simulink model "cochons_optim"  (R2013b)
settings: Solver=ode45  StartTime=0  StopTime=12000  RelTol=1e-3
libraries: simulink x3
settings Model: TunableVars=p  TunableVarsStorageClass=Auto  Creator=ltraonou  LastModifiedBy=ltraonou
settings SolverCC: ShapePreserveControl=EnableAll
settings DataIOCC: FinalStateName=last_state  InitialState=last_state  LimitDataPoints=off  SaveFormat=StructureWithTime  SaveOutput=off  SaveTime=off
settings OptimizationCC: InlineParams=on
settings DebuggingCC: MultiTaskDSMMsg=warning  MultiTaskCondExecSysMsg=none
settings RTWCC: IncludeERTFirstTime=on

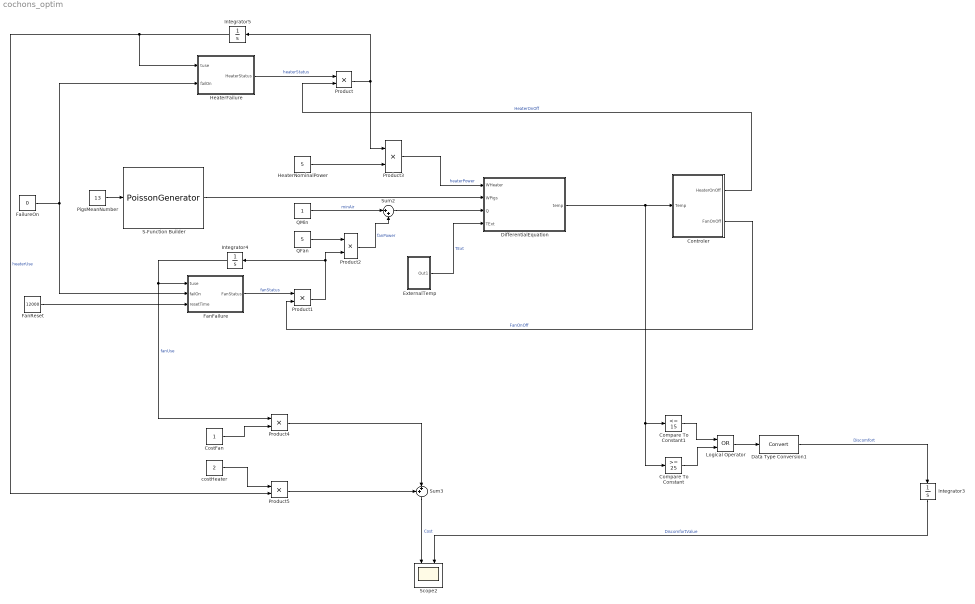
== system cochons_optim ==
  Compare To Constant : simulink/Logic and Bit Operations/Compare To Constant  relop=>=  const=25  OutDataTypeStr=boolean
  Compare To Constant1 : simulink/Logic and Bit Operations/Compare To Constant  relop=<=  const=15  OutDataTypeStr=boolean
  Controler : Subsystem
  CostFan : Constant
  Data Type Conversion1 : DataTypeConversion
  DifferentialEquation : Subsystem
  ExternalTemp : Subsystem
  FailureOn : Constant  Value=0
  FanFailure : Subsystem
  FanReset : Constant  Value=12000
  HeaterFailure : Subsystem
  HeaterNominalPower : Constant  Value=5
  Integrator3 : Integrator  InitialCondition=0.0001
  Integrator4 : Integrator
  Integrator5 : Integrator
  Logical Operator : Logic  Operator=OR  AllPortsSameDT=off  OutDataTypeStr=boolean
  PigsMeanNumber : Constant  Value=13
  Product{,1..5} (6 alike) : Product
  QFan : Constant  Value=5
  QMin : Constant
  S-Function Builder : S-Function  InitFcn=try, set_param(gcb,'FunctionName','PoissonGenerator'), end  FunctionName=PoissonGenerator  SFunctionModules=PoissonGenerator_wrapper  EnableBusSupport=off  mask(S-Function Builder){}
      mask help: Simulink:masks:SFunctionBuilder_MD
      mask init:
      | val = [[.9  0.75 0.75 1 1 .9 .9 1]',[1 1 0.75 0.75 .9 .9 1 .9]'];try , sys = get_param(gcb,'SfunBuilderFcnName');if isempty(sys), sys = get_param(gcb,'FunctionName'); end,catch, sys = get_param(gcb,'FunctionName'); end
      settings: CopyFcn=set_param(gcbh,'LinkStatus','none')  PreSaveFcn=try, set_param(gcb,'FunctionName','PoissonGenerator'), end  OpenFcn=sfunctionwizard(gcbh)
      mask Display: plot(val(:,1),val(:,2)),disp(sys), port_label('input',1,'lambda'), port_label('output',1,'y')
  Scope2 : Scope  NumInputPorts=2
      settings: YMin=0~0  YMax=7500~325
  Sum2 : Sum  Inputs=|++
  Sum3 : Sum  Inputs=++|
  costHeater : Constant  Value=2
  wires:
  QFan/1 -> Product2/1
  QMin/1 -> Sum2/1  "minAir"
  Product2/1 -> Sum2/2  "fanPower"
  Product3/1 -> DifferentialEquation/1(WHeater)  "heaterPower"
  HeaterNominalPower/1 -> Product3/2
  FanFailure/1(FanStatus) -> Product1/1  "fanStatus"
  HeaterFailure/1(HeaterStatus) -> Product/1  "heaterStatus"
  Controler/2(FanOnOff) -> Product1/2  "FanOnOff"
  Controler/1(HeaterOnOff) -> Product/2  "HeaterOnOff"
  Data Type Conversion1/1 -> Integrator3/1  "Discomfort"
  DifferentialEquation/1(temp) -> Controler/1(Temp), Compare To Constant/1, Compare To Constant1/1
  S-Function Builder/1 -> DifferentialEquation/2(WPigs)
  Sum2/1 -> DifferentialEquation/3(Q)
  PigsMeanNumber/1 -> S-Function Builder/1
  ExternalTemp/1(Out1) -> DifferentialEquation/4(TExt)  "TExt"
  Compare To Constant1/1 -> Logical Operator/1
  Compare To Constant/1 -> Logical Operator/2
  Logical Operator/1 -> Data Type Conversion1/1
  Product/1 -> Integrator5/1, Product3/1
  Product1/1 -> Product2/2, Integrator4/1
  FailureOn/1 -> HeaterFailure/2(failOn), FanFailure/2(failOn)
  FanReset/1 -> FanFailure/3(resetTime)
  Integrator3/1 -> Scope2/2  "DiscomfortValue"
  CostFan/1 -> Product4/2
  Product4/1 -> Sum3/2
  Sum3/1 -> Scope2/1  "Cost"
  Integrator4/1 -> Product4/1, FanFailure/1(tuse)  "fanUse"
  Integrator5/1 -> HeaterFailure/1(tuse), Product5/2  "heaterUse"
  costHeater/1 -> Product5/1
  Product5/1 -> Sum3/1

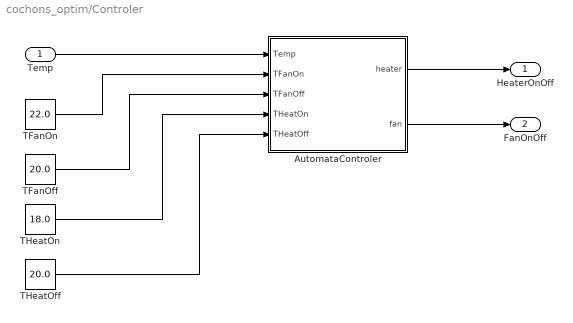
== system cochons_optim/Controler ==
  Temp : Inport
  AutomataControler : Stateflow chart  TreatAsAtomicUnit=on
  TFanOff : Constant  Value=20.0
  TFanOn : Constant  Value=22.0
  THeatOff : Constant  Value=20.0
  THeatOn : Constant  Value=18.0
  HeaterOnOff : Outport
  FanOnOff : Outport  Port=2
  wires:
  Temp/1 -> AutomataControler/1(Temp)
  TFanOn/1 -> AutomataControler/2(TFanOn)
  THeatOn/1 -> AutomataControler/4(THeatOn)
  THeatOff/1 -> AutomataControler/5(THeatOff)
  TFanOff/1 -> AutomataControler/3(TFanOff)
  AutomataControler/2(fan) -> FanOnOff/1
  AutomataControler/1(heater) -> HeaterOnOff/1

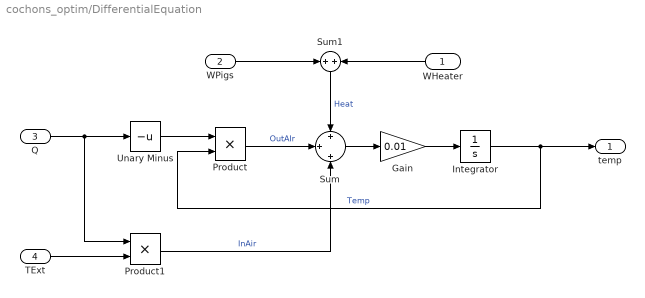
== system cochons_optim/DifferentialEquation ==
  WHeater : Inport
  WPigs : Inport  Port=2
  Q : Inport  Port=3
  TExt : Inport  Port=4
  Gain : Gain  Gain=0.01
  Integrator : Integrator  InitialCondition=20
  Product : Product
  Product1 : Product
  Sum : Sum  Inputs=+|+|+
  Sum1 : Sum  Inputs=+|+
  Unary Minus : UnaryMinus
  temp : Outport
  wires:
  WHeater/1 -> Sum1/2
  Sum1/1 -> Sum/1  "Heat"
  Unary Minus/1 -> Product/1
  Product1/1 -> Sum/3  "InAir"
  Product/1 -> Sum/2  "OutAIr"
  Q/1 -> Product1/1, Unary Minus/1
  Sum/1 -> Gain/1
  Gain/1 -> Integrator/1
  WPigs/1 -> Sum1/1
  Integrator/1 -> Product/2, temp/1  "Temp"
  TExt/1 -> Product1/2

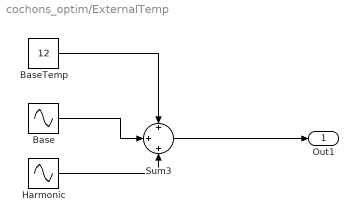
== system cochons_optim/ExternalTemp ==
  Base : Sin  Amplitude=10  Frequency=0.01  SampleTime=0
  BaseTemp : Constant  Value=12
  Harmonic : Sin  Amplitude=3  Frequency=0.1  SampleTime=0
  Sum3 : Sum  Inputs=+|+|+
  Out1 : Outport
  wires:
  BaseTemp/1 -> Sum3/1
  Sum3/1 -> Out1/1
  Base/1 -> Sum3/2
  Harmonic/1 -> Sum3/3

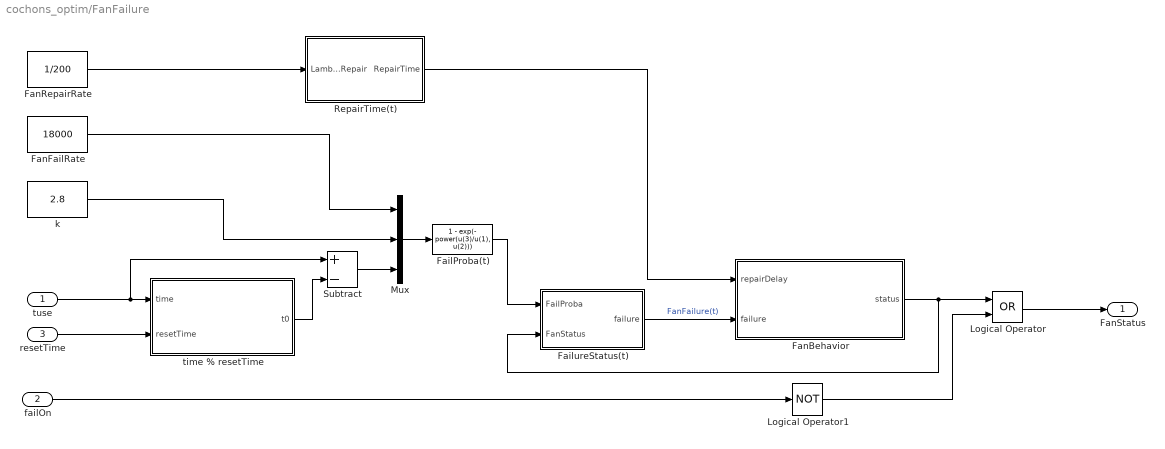
== system cochons_optim/FanFailure ==
  tuse : Inport
  failOn : Inport  Port=2
  resetTime : Inport  Port=3
  FailProba(t) : Fcn  Expr=1 - exp(- power(u(3)/u(1), u(2)))
  FailureStatus(t) : Subsystem
  FanBehavior : Stateflow chart  TreatAsAtomicUnit=on
  FanFailRate : Constant  Value=18000
  FanRepairRate : Constant  Value=1/200
  Logical Operator : Logic  Operator=OR  AllPortsSameDT=off  OutDataTypeStr=boolean
  Logical Operator1 : Logic  Operator=NOT  AllPortsSameDT=off  OutDataTypeStr=boolean
  Mux : Mux  Inputs=3
  RepairTime(t) : Subsystem
  Subtract : Sum  Inputs=+-
  k : Constant  Value=2.8
  time % resetTime : Stateflow chart  TreatAsAtomicUnit=on
  FanStatus : Outport
  wires:
  failOn/1 -> Logical Operator1/1
  Logical Operator1/1 -> Logical Operator/2
  FanBehavior/1(status) -> FailureStatus(t)/2(FanStatus), Logical Operator/1
  Logical Operator/1 -> FanStatus/1
  FanRepairRate/1 -> RepairTime(t)/1(LambdaRepair)
  time % resetTime/1(t0) -> Subtract/2
  resetTime/1 -> time % resetTime/2(resetTime)
  Mux/1 -> FailProba(t)/1
  FailProba(t)/1 -> FailureStatus(t)/1(FailProba)
  RepairTime(t)/1(RepairTime) -> FanBehavior/1(repairDelay)
  Subtract/1 -> Mux/3
  k/1 -> Mux/2
  tuse/1 -> Subtract/1, time % resetTime/1(time)
  FailureStatus(t)/1(failure) -> FanBehavior/2(failure)  "FanFailure(t)"
  FanFailRate/1 -> Mux/1

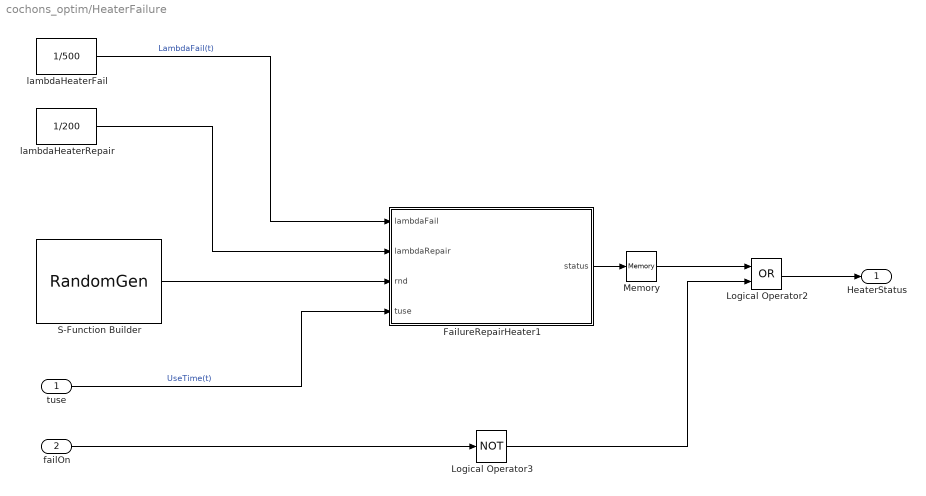
== system cochons_optim/HeaterFailure ==
  tuse : Inport
  failOn : Inport  Port=2
  FailureRepairHeater1 : Stateflow chart  TreatAsAtomicUnit=on
  Logical Operator2 : Logic  Operator=OR  AllPortsSameDT=off  OutDataTypeStr=boolean
  Logical Operator3 : Logic  Operator=NOT  AllPortsSameDT=off  OutDataTypeStr=boolean
  Memory : Memory
  S-Function Builder : S-Function  InitFcn=try, set_param(gcb,'FunctionName','RandomGen'), end  FunctionName=RandomGen  SFunctionModules=RandomGen_wrapper  EnableBusSupport=off  mask(S-Function Builder){}
      mask help: Simulink:masks:SFunctionBuilder_MD
      mask init: same as cochons_optim/S-Function Builder
      settings: CopyFcn=set_param(gcbh,'LinkStatus','none')  PreSaveFcn=try, set_param(gcb,'FunctionName','RandomGen'), end  OpenFcn=sfunctionwizard(gcbh)
      mask Display: plot(val(:,1),val(:,2)),disp(sys), port_label('output',1,'y0')
  lambdaHeaterFail : Constant  Value=1/500
  lambdaHeaterRepair : Constant  Value=1/200
  HeaterStatus : Outport
  wires:
  lambdaHeaterRepair/1 -> FailureRepairHeater1/2(lambdaRepair)
  S-Function Builder/1 -> FailureRepairHeater1/3(rnd)
  FailureRepairHeater1/1(status) -> Memory/1
  failOn/1 -> Logical Operator3/1
  Logical Operator3/1 -> Logical Operator2/2
  tuse/1 -> FailureRepairHeater1/4(tuse)  "UseTime(t)"
  Logical Operator2/1 -> HeaterStatus/1
  lambdaHeaterFail/1 -> FailureRepairHeater1/1(lambdaFail)  "LambdaFail(t)"
  Memory/1 -> Logical Operator2/1

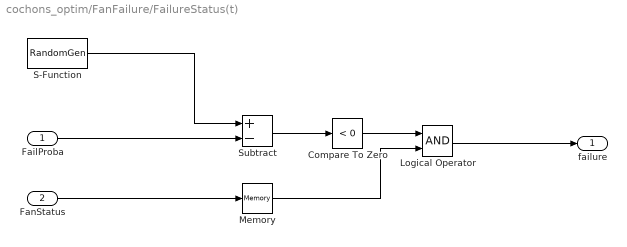
== system cochons_optim/FanFailure/FailureStatus(t) ==
  FailProba : Inport
  FanStatus : Inport  Port=2
  Compare To Zero : simulink/Logic and Bit Operations/Compare To Zero  relop=<  OutDataTypeStr=boolean
  Logical Operator : Logic  AllPortsSameDT=off  OutDataTypeStr=boolean
  Memory : Memory
  S-Function : S-Function  FunctionName=RandomGen  EnableBusSupport=off
  Subtract : Sum  Inputs=+-
  failure : Outport
  wires:
  S-Function/1 -> Subtract/1
  FailProba/1 -> Subtract/2
  Subtract/1 -> Compare To Zero/1
  FanStatus/1 -> Memory/1
  Compare To Zero/1 -> Logical Operator/1
  Logical Operator/1 -> failure/1
  Memory/1 -> Logical Operator/2

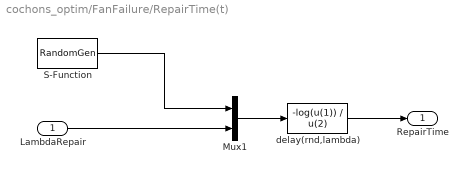
== system cochons_optim/FanFailure/RepairTime(t) ==
  LambdaRepair : Inport
  Mux1 : Mux  Inputs=2
  S-Function : S-Function  FunctionName=RandomGen  EnableBusSupport=off
  delay(rnd,lambda) : Fcn  Expr=-log(u(1)) / u(2)
  RepairTime : Outport
  wires:
  Mux1/1 -> delay(rnd,lambda)/1
  LambdaRepair/1 -> Mux1/2
  delay(rnd,lambda)/1 -> RepairTime/1
  S-Function/1 -> Mux1/1

== stateflow chart cochons_optim/FanFailure/FanBehavior ==
  state Failure
    status=0;
    delay=repairDelay;
  state Ok
    status=1;
  Failure -> Ok : [after(delay,sec)]
  (default) -> Ok
  Ok -> Failure : [failure]
  data: status output double; repairDelay input; failure input; delay local double

== stateflow chart cochons_optim/Controler/AutomataControler ==
  state Idle
    heater=0;
    fan=0;
  state Fan_on
    heater=0;
    fan=1;
  state Heater_on
    heater=1;
    fan=0;
  (default) -> Idle
  Fan_on -> Idle : [Temp<=TFanOff]
  Idle -> Fan_on [order 1] : [Temp>=TFanOn]
  Idle -> Heater_on [order 2] : [Temp<=THeatOn]
  Heater_on -> Idle : [Temp>=THeatOff]
  data: heater output double; Temp input; fan output double; TFanOn input; TFanOff input; THeatOn input; THeatOff input

== stateflow chart cochons_optim/HeaterFailure/FailureRepairHeater1 ==
  state Repair_After_trepair
  state Failure
    status=0;
    trepair=-log(rnd)/lambdaRepair;
  state Ok
    status=1;
    tfail=(-log(rnd)/lambdaFail)+tuse;
  state Fail_After_tfail
  Repair_After_trepair -> Ok : [after(trepair,sec)]
  Failure -> Repair_After_trepair
  (default) -> Ok
  Ok -> Fail_After_tfail
  Fail_After_tfail -> Failure : [tuse>=tfail]
  data: lambdaFail input; status output double; lambdaRepair input; rnd input; tfail local double; trepair local double; tuse input

== stateflow chart cochons_optim/FanFailure/time % resetTime ==
  state WAIT
  state RESET
  (default) -> WAIT : {t0 = time;}
  RESET -> WAIT : {t0 = time;}
  WAIT -> RESET : [after(resetTime,sec)]
  data: time input; resetTime input double; t0 output double =0
